simulink model "CDMA2000sint_C_etapa2"  (R2012b)
settings: Solver=ode45  StartTime=0.0  StopTime=10.0  RelTol=1e-3
libraries: commcnvcod2 x2, commrandsrc2 x1
settings Model: Creator=student  LastModifiedBy=student

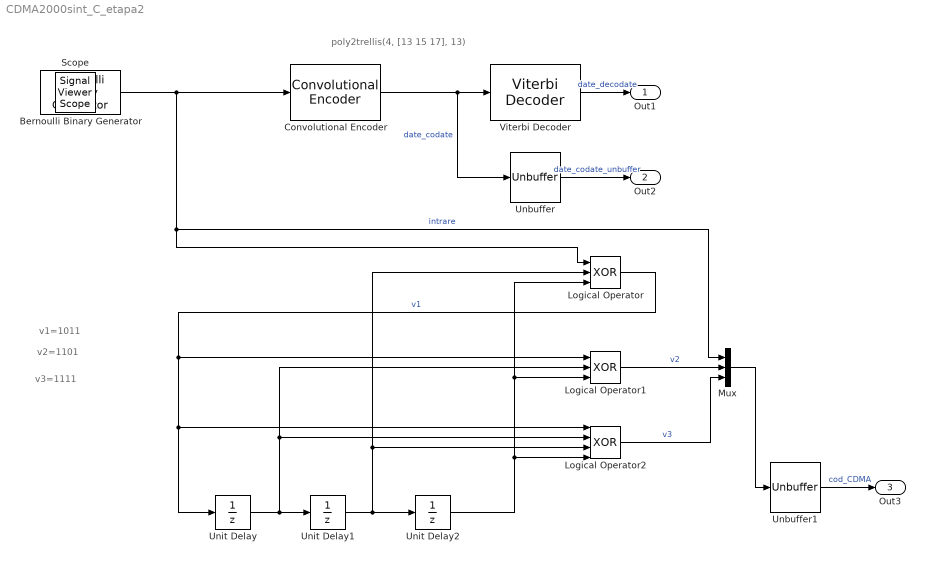
== system CDMA2000sint_C_etapa2 ==
  note: v3=1111
  note: v2=1101
  note: v1=1011
  note: poly2trellis(4, [13 15 17], 13)
  Bernoulli Binary Generator : commrandsrc2/Bernoulli Binary Generator  P=0.5  seed=61  Ts=1  frameBased=off  sampPerFrame=1  orient=off  outDataType=boolean
  Convolutional Encoder : commcnvcod2/Convolutional Encoder  trellis=poly2trellis(4, [13 15 17], 13)  opMode=Continuous  DelayedResetAction=off  hasIniStPort=off  hasFinStPort=off  usePuncVector=off  punctureVector=[1; 1; 0; 1; 0; 1]  reset=Unused parameter value
  Logical Operator : Logic  Operator=XOR  Inputs=3  IconShape=distinctive  AllPortsSameDT=off  OutDataTypeStr=boolean
  Logical Operator1 : Logic  Operator=XOR  Inputs=3  IconShape=distinctive  AllPortsSameDT=off  OutDataTypeStr=boolean
  Logical Operator2 : Logic  Operator=XOR  Inputs=4  IconShape=distinctive  AllPortsSameDT=off  OutDataTypeStr=boolean
  Mux : Mux  Inputs=3
  Unbuffer : Unbuffer  SampleBasedProcessing=Same as frame based
  Unbuffer1 : Unbuffer  SampleBasedProcessing=Same as frame based
  Unit Delay : UnitDelay  SampleTime=-1
  Unit Delay1 : UnitDelay  SampleTime=-1
  Unit Delay2 : UnitDelay  SampleTime=-1
  Viterbi Decoder : commcnvcod2/Viterbi Decoder  trellis=poly2trellis(4, [13 15 17], 13)  isPunctured=off  punctureVector=[1; 1; 0; 1; 0; 1]  erasures=off  dectype=Hard decision  runSigValErrCheck=off  nsdecb=4  smWordLength=16  tbdepth=1  opmode=Continuous  reset=off  outDataType=boolean  delayedResetAction=off
  Out1 : Outport
  Out2 : Outport  Port=2
  Out3 : Outport  Port=3
  Scope : SignalViewerScope  IOType=viewer  NumInputPorts=4  RefreshTime=0.035000
      settings: ShowDataMarkers=on  YMin=-5~-5~-5~-5  YMax=5~5~5~5
  wires:
  Bernoulli Binary Generator/1 -> Mux/1, Logical Operator/1, Convolutional Encoder/1  "intrare"
  Convolutional Encoder/1 -> Unbuffer/1, Viterbi Decoder/1  "date_codate"
  Viterbi Decoder/1 -> Out1/1  "date_decodate"
  Unbuffer/1 -> Out2/1  "date_codate_unbuffer"
  Logical Operator/1 -> Logical Operator1/1, Logical Operator2/1, Unit Delay/1  "v1"
  Unit Delay/1 -> Logical Operator1/2, Logical Operator2/2, Unit Delay1/1
  Unit Delay1/1 -> Logical Operator/2, Logical Operator2/3, Unit Delay2/1
  Unit Delay2/1 -> Logical Operator1/3, Logical Operator/3, Logical Operator2/4
  Logical Operator1/1 -> Mux/2  "v2"
  Logical Operator2/1 -> Mux/3  "v3"
  Mux/1 -> Unbuffer1/1
  Unbuffer1/1 -> Out3/1  "cod_CDMA"
